simulink model "prova"  (Simulink 7.4)
settings: Solver=ode45  StartTime=0.0  StopTime=10.0  RelTol=1e-3
libraries: roblocks x4
settings Model: Creator=acolome  LastModifiedBy=acolome

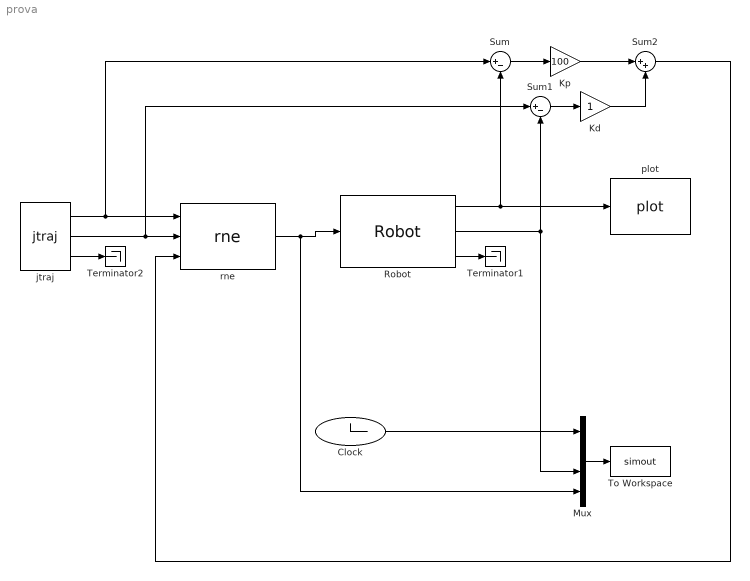
== system prova ==
  Clock : Clock
      settings: Decimation=10
  Kd : Gain  SaturateOnIntegerOverflow=on  OutDataTypeStr=Inherit: Same as input  ParamDataTypeStr=Inherit: Same as input
  Kp : Gain  Gain=100  SaturateOnIntegerOverflow=on  OutDataTypeStr=Inherit: Same as input  ParamDataTypeStr=Inherit: Same as input
  Mux : Mux
  Robot : roblocks/Robot  SystemSampleTime=-1  robot=p560  q0=[0 0 0 0 0 0]
  Sum : Sum  Inputs=|+-  SaturateOnIntegerOverflow=on  InputSameDT=on  OutDataTypeStr=Inherit: Same as first input
  Sum1 : Sum  Inputs=|+-  SaturateOnIntegerOverflow=on  InputSameDT=on  OutDataTypeStr=Inherit: Same as first input
  Sum2 : Sum  Inputs=|++  SaturateOnIntegerOverflow=on  InputSameDT=on  OutDataTypeStr=Inherit: Same as first input
  Terminator1 : Terminator
  Terminator2 : Terminator
  To Workspace : ToWorkspace  VariableName=simout  SampleTime=-1  SaveFormat=Array
  jtraj : roblocks/jtraj  SystemSampleTime=-1  q0=[0 0 0 0 0 0]  qf=[pi/4 pi/2 -pi/2 0 0 0]  tmax=5
      link override MATLAB Fcn: MATLABFcn=squeeze(interp1(t,q,u))
      link override MATLAB Fcn1: MATLABFcn=squeeze(interp1(t,qd,u))
      link override MATLAB Fcn2: MATLABFcn=squeeze(interp1(t,qdd,u))
  plot : roblocks/plot  SystemSampleTime=-1  robot=p560
  rne : roblocks/rne  SystemSampleTime=-1  robot=p560  grav=[0 0 9.81]
  wires:
  ? -> ?
  jtraj/1 -> rne/1, Sum/1
  jtraj/2 -> rne/2, Sum1/1
  Robot/2 -> Mux/3, Sum1/2
  Robot/3 -> Terminator1/1
  Mux/1 -> To Workspace/1
  Clock/1 -> Mux/1
  jtraj/3 -> Terminator2/1
  rne/1 -> Robot/1, Mux/4
  Sum/1 -> Kp/1
  Kp/1 -> Sum2/1
  Sum1/1 -> Kd/1
  Kd/1 -> Sum2/2
  Sum2/1 -> rne/3
  Robot/1 -> plot/1, Sum/2
